simulink model "ANDChart"  (R2023a)
settings: Solver=VariableStepAuto  StartTime=0.0  StopTime=10.0  RelTol=1e-3
settings Model: Creator=Egypt_Laptop  LastModifiedBy=Egypt_Laptop

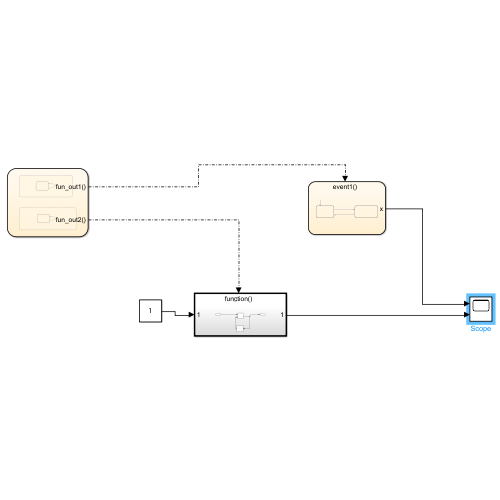
[thumbnail: Simulink's stored preview of the top-level diagram]
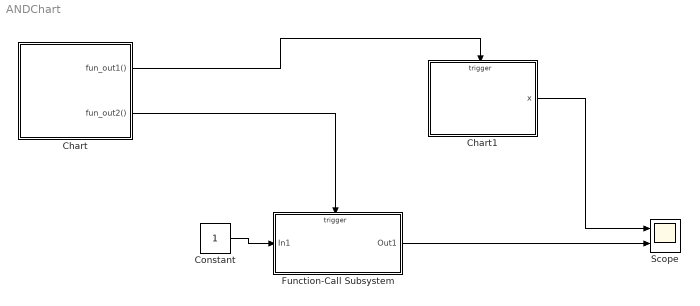
== system ANDChart ==
  Chart : Stateflow chart  TreatAsAtomicUnit=on
  Chart1 : Stateflow chart  TreatAsAtomicUnit=on
  Constant : Constant
  Function-Call Subsystem : Subsystem  TreatAsAtomicUnit=on
  Scope : Scope  NumInputPorts=2
  wires:
  Function-Call Subsystem/1(Out1) -> Scope/2
  Constant/1 -> Function-Call Subsystem/1(In1)
  Chart/2(fun_out2()) -> Function-Call Subsystem/Trigger
  Chart1/1(x) -> Scope/1
  Chart/1(fun_out1()) -> Chart1/Trigger

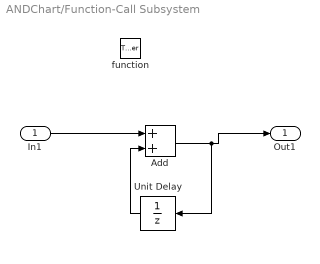
== system ANDChart/Function-Call Subsystem ==
  In1 : Inport
  function : TriggerPort  TriggerType=function-call  VariantControl=(inherit)
  Add : Sum
  Unit Delay : UnitDelay  SampleTime=-1  HasFrameUpgradeWarning=on
  Out1 : Outport
  wires:
  Add/1 -> Unit Delay/1, Out1/1
  In1/1 -> Add/1
  Unit Delay/1 -> Add/2

== stateflow chart ANDChart/Chart1 ==
  settings: executeAtInitialization=1
  state s1
    en: x=0;
  state s2
    en: x=1;
  (default) -> s1
  s1 -> s2
  s2 -> s1
  data: x output
  events: event1 input FUNCTION_CALL_EVENT

== stateflow chart ANDChart/Chart ==
  state A1 [parallel]
    settings: executionOrder=1
    state S1
    S1 -> S1 : after(0.5,sec){fun_out1}
  state A2 [parallel]
    settings: executionOrder=2
    state S2
    S2 -> S2 : after(0.5,sec){fun_out2}
  events: fun_out1 output FUNCTION_CALL_EVENT; fun_out2 output FUNCTION_CALL_EVENT
